simulink model "statespacejahdskjsdhkad"  (R2018a)
settings: Solver=VariableStepAuto  StartTime=0.0  StopTime=10.0  RelTol=1e-3
values from neighbouring files (symbols this model uses):
  A = [-(a1/A1), 0; a1*A1, -(a2/A2)]    [linearyzacjamud6.m]
  A1 = 1    [linearyzacjamud6.m]
  a1 = Aw1*sqrt(2*g)    [linearyzacjamud6.m]
  B = [1/A1; 0]    [linearyzacjamud6.m]
  C = [1,0;0,1]    [linearyzacjamud6.m]
  D = [0;0]    [linearyzacjamud6.m]
  fwe = 0.9*fwemax    [linearyzacjamud6.m]
  IC = [h1pocz;h2pocz]    [linearyzacjamud6.m]
settings Model: Creator=john  LastModifiedBy=john

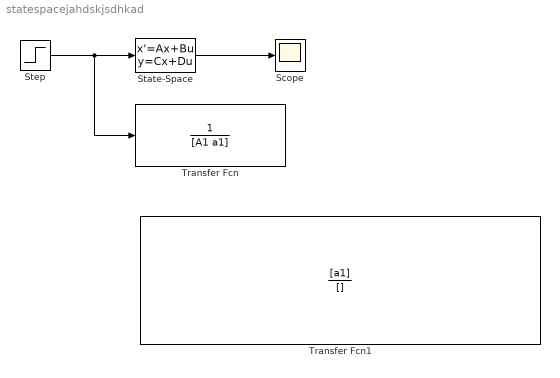
== system statespacejahdskjsdhkad ==
  Scope : Scope
  State-Space : StateSpace  A=A  B=B  C=C  D=D  InitialCondition=IC
  Step : Step  Time=0  After=fwe  SampleTime=0
  Transfer Fcn : TransferFcn  Denominator=[A1 a1]
  Transfer Fcn1 : TransferFcn  Numerator=[a1]  Denominator=[]
  wires:
  Step/1 -> Transfer Fcn/1, State-Space/1
  State-Space/1 -> Scope/1
